simulink model "master_thesis_simulink"  (R2022a)
settings: Solver=VariableStepAuto  StartTime=0.0  StopTime=p_0p.time(end)  FixedStep=0.001  RelTol=1e-3
values from neighbouring files (symbols this model uses):
  markers_forearm = [0.00210510253906 -0.143263397217 -0.00798474121094]    [markers_forearm.mat]
  markers_shoulder = [0.010127746582 -0.151647644043 -0.0119686279297]    [markers_shoulder.mat]
undefined symbols (not defined in the file or in its folder): arm, DiscIntNeverNeededParam, Discrete, ekf, kf, LS, m, markers_hand, n, noise, q0, q0_LS, q0_model, sample_Time, selected, state_observer, Time, tSh_0_0Conf, X, Y, Z
libraries: sm_lib x2029, nesl_utility x1553, robotlib x75, ctrlSharedLib x8
(part 2 of 70)

== system master_thesis_simulink/System/Human arm ==
  note: B_shoulder
  note: SHOULDER
  note: ELBOW-FOREARM
  note: WRIST-HAND
  q ref : Inport
  Demux : Demux  Outputs=7
  Elbow_joint : Subsystem
      settings: PortSchema="{\"entries\":[{\"content\":{\"sides\":[{\"content\":{\"connectorIds\":[\"LConn1\",\"In1\"]},\"type\":\"ConnectorPlacement.EquallySpacedRectSide\",\"uuid\":\"7172d894-cd28-4181-98d4-69e790c9ffe7\"},{\"content\":{\"connectorIds\":[\"RConn1\"],\"side\":\"RIGHT\"},\"type\":\"ConnectorPlacement.EquallySpacedRectSide\",\"uuid\":\"72334abd-f6e9-45ab-9ec0-c8814621d72e\"},{\"content\":{\"connectorIds\":[],\"side\":\"TOP\"},\"type\":\"ConnectorPlacement.EquallySpacedRectSide\",\"uuid\":\"097d2b6b-6630-427f-97b0-bc88c7b983e5\"}]},\"type\":\"ConnectorPlacement.EquallySpacedConnector\",\"uuid\":\"52d59dae-be5f-4018-861b-6a79689710e1\"}],\"packageUris\":[\"http://schema.mathworks.com/mf0/Connector/R2020b\"],\"version\":\"1.0\"}"
  Markers : Subsystem  Commented=on
  Mechanism Configuration : sm_lib/Utilities/Mechanism Configuration  UniformGravity=Constant  GravityVector=[0 0 -9.80665]  GravityUnits=m/s^2  LinearizationDelta=0.001  JointModeTransitionNonlinearIterations=2
  Mux : Mux  Inputs=m
  Mux1 : Mux  Inputs=m
  Mux2 : Mux  Inputs=3
  Mux3 : Mux  Inputs=3
  RightForeArm : Subsystem
  RightHand : Subsystem
  RightShoulder : Subsystem
  RightShoulder_joint : Subsystem
      settings: PortSchema="{\"entries\":[{\"content\":{\"sides\":[{\"content\":{\"connectorIds\":[\"LConn1\",\"In1\"]},\"type\":\"ConnectorPlacement.EquallySpacedRectSide\",\"uuid\":\"7172d894-cd28-4181-98d4-69e790c9ffe7\"},{\"content\":{\"connectorIds\":[\"RConn1\"],\"side\":\"RIGHT\"},\"type\":\"ConnectorPlacement.EquallySpacedRectSide\",\"uuid\":\"72334abd-f6e9-45ab-9ec0-c8814621d72e\"},{\"content\":{\"connectorIds\":[],\"side\":\"TOP\"},\"type\":\"ConnectorPlacement.EquallySpacedRectSide\",\"uuid\":\"097d2b6b-6630-427f-97b0-bc88c7b983e5\"}]},\"type\":\"ConnectorPlacement.EquallySpacedConnector\",\"uuid\":\"52d59dae-be5f-4018-861b-6a79689710e1\"}],\"packageUris\":[\"http://schema.mathworks.com/mf0/Connector/R2020b\"],\"version\":\"1.0\"}"
  Solver Configuration1 : nesl_utility/Solver Configuration  PhysicalDomain=network_engine_domain  SubClassName=solver  LeftPortType=input  RightPortType=generic  Tones=[]  Harmonics=[]  SimulateNoise=off  Profile=off  UseLocalSampling=off  EnableSwitchedLinearOptims=on  FrequencyDomain=off  UseCCode=off  RelTol=0.001  AbsTol=0.001  MinStep=1e-09  ToWorkspace=off  RevertToSquareIcSolve=off  NumHomotopyIterations=100  PhasorMode=off  PhasorModeNumHarmonics=1  IndexReductionMethod=DerivativeReplacement  DoDC=off  ResidualTolerance=1e-09  UseLocalSolver=off  LocalSolverChoice=NE_BACKWARD_EULER_ADVANCER  LocalSolverSampleTime=0.001  DoFixedCost=off  MaxNonlinIter=3  MaxModeIter=2  ComputeImpulses=off  ImpulseIterations=2  LinearAlgebra=auto  LinearAlgebraNumThread=0  EquationFormulation=NE_TIME_EF  DelaysMemoryBudget=1024  AutomaticFiltering=on  FilteringTimeConstant=0.001  PartitionStorageMethod=AS_NEEDED  PartitionMemoryBudget=1024  PartitionMethod=ROBUST
      settings: SourceProductBaseCode=SS,PW,VE
  World Frame : sm_lib/Frames and Transforms/World Frame
  Wrist_joint : Subsystem
  p : Outport
  pdot : Outport  Port=2
  wires:
  Mux/1 -> p/1
  Mux1/1 -> pdot/1
  q ref/1 -> Demux/1
  Demux/7 -> Mux3/3
  Demux/1 -> Mux2/1
  Demux/2 -> Mux2/2
  Demux/3 -> Mux2/3
  Demux/6 -> Mux3/2
  Demux/5 -> Mux3/1
  Demux/4 -> [q_El]
  Mux2/1 -> [q_Sh]
  Mux3/1 -> [q_Wr]
  [q_Sh] -> RightShoulder_joint/1(q ref 1..3)
  [q_Wr] -> Wrist_joint/1(q ref 5..7)
  [q_El] -> Elbow_joint/1(q ref 4)
  [p_1] -> Mux/1
  [pdot_1] -> Mux1/1
  [p_2] -> Mux/2
  [pdot_2] -> Mux1/2
  [p_3] -> Mux/3
  [pdot_3] -> Mux1/3
  connections:
  RightShoulder/LConn1 -- RightShoulder_joint/RConn1
  RightHand/LConn1 -- Wrist_joint/RConn1
  Elbow_joint/LConn1 -- RightShoulder/RConn1
  RightForeArm/LConn2 -- RightHand/LConn2 -- RightShoulder/LConn2 -- World Frame/RConn1 -- RightShoulder_joint/LConn1 -- Mechanism Configuration/RConn1 -- Solver Configuration1/RConn1
  Elbow_joint/RConn1 -- RightForeArm/LConn1
  RightForeArm/RConn1 -- Wrist_joint/LConn1

== system master_thesis_simulink/System/LKF ==
  pdot_k : Inport
  p_k : Inport  Port=2
  Kalman Filter : MATLAB Function  TreatAsAtomicUnit=on
  Kalman Filter1 : ctrlSharedLib/Kalman Filter  Commented=on  TimeDomain=Discrete-Time  UseCurrentEstimator=on  ModelSource=Individual A, B, C, D matrices  ModelSourceVariable=ss(0.95,1,1,0,1)  A=kf.F  B=kf.G  C=kf.J  D=kf.I  NumberOfStates=1  NumberOfInputs=1  NumberOfOutputs=1  InitialEstimateSource=Dialog  X0=kf.Delta_q0  P0=kf.P0  UseK=off  UseGH=off  NumberOfProcessNoiseInputs=1  G=1  TimeInvariantG=on  H=0  TimeInvariantH=on  Q=noise.Q  TimeInvariantQ=on  R=noise.R  TimeInvariantR=on  N=0  TimeInvariantN=on  AddInputPort=on  AddEnablePort=off  OutputEstimatedY=off  OutputP=off  Ts=sample_Time
  Saturation : Saturate  UpperLimit=[pi/2; pi/10; 2/3*pi; pi/2; pi/4; pi/10; pi/4]  LowerLimit="[-pi/2; -pi/10; -pi/6; 0; -pi/2;  -pi/2; -pi/4]"
  Scope : Scope  NumInputPorts=2
  Sum2 : Sum  Inputs=++|
  Sum3 : Sum  Inputs=|+-
  Sum4 : Sum  Inputs=++|
  Sum6 : Sum  Inputs=|+-
  To Workspace1 : ToWorkspace  VariableName=q_KF  SaveFormat=Structure With Time  SampleTime=-1
  p_eq : Constant  Value=kf.p_eq  SampleTime=sample_Time
  pdot_eq : Constant  Value=kf.pdot_eq  SampleTime=sample_Time
  q_eq : Constant  Value=kf.q_eq  SampleTime=sample_Time
  q_eq1 : Constant  Value=kf.q_eq  SampleTime=sample_Time
  q_KF : Outport
  wires:
  pdot_k/1 -> Sum3/1
  pdot_eq/1 -> Sum3/2
  Sum3/1 -> Kalman Filter1/1, Kalman Filter/2(Delta_pdotk_1)
  Kalman Filter/1(Delta_qk) -> Sum2/2
  Kalman Filter1/1 -> Sum4/2
  q_eq1/1 -> Sum4/1
  Sum4/1 -> Scope/2  "kf simulink"
  p_k/1 -> Sum6/1
  p_eq/1 -> Sum6/2  "u_eqk"
  Sum6/1 -> Kalman Filter1/2, Kalman Filter/1(Delta_pk)  "Delta_uk"
  q_eq/1 -> Sum2/1
  Sum2/1 -> Saturation/1  "kf"
  Saturation/1 -> To Workspace1/1, q_KF/1, Scope/1

== system master_thesis_simulink/System/LS ==
  pdot : Inport
  Integrator : Integrator  InitialCondition=q0_LS  LimitOutput=on  UpperSaturationLimit=[pi/2; pi/10; 2/3*pi; pi/2; pi/4; pi/10; pi/4]  LowerSaturationLimit="[-pi/2; -pi/10; -pi/6; 0; -pi/2;  -pi/2; -pi/4]"
  LS : MATLAB Function  TreatAsAtomicUnit=on
  To Workspace1 : ToWorkspace  VariableName=q_LS_MinimumNorm  SaveFormat=Structure With Time  SampleTime=-1
  q_LS : Outport
  tag scope: q_LS_MinimumNorm=global
  wires:
  [markers_s] -> LS/3(shoulder_variables)
  [markers_h] -> LS/5(hand_variables)
  [markers_f] -> LS/4(forearm_variables)
  pdot/1 -> LS/2(pdot)
  [q_LS_MinimumNorm] -> LS/1(q_LS_MinimumNorm)
  Integrator/1 -> To Workspace1/1, q_LS/1, [q_LS_MinimumNorm]  "q_LS_MinimumNorm"
  LS/1(qdot_LS_MinimumNorm) -> Integrator/1

== system master_thesis_simulink/System/Noisy p ==
  p_true : Inport
  Sum1 : Sum  Inputs=++|
  v : RandomNumber  Variance=diag(noise.R)  Seed=2  SampleTime=sample_Time
  p : Outport
  wires:
  p_true/1 -> Sum1/2
  Sum1/1 -> p/1  "p"
  v/1 -> Sum1/1

== system master_thesis_simulink/System/Noisy pdot ==
  pdot_true : Inport
  Sum1 : Sum  Inputs=++|
  n_pdot : RandomNumber  Variance=diag(noise.N_pdot)  Seed=2  SampleTime=sample_Time
  pdot : Outport
  wires:
  pdot_true/1 -> Sum1/2
  Sum1/1 -> pdot/1  "pdot"
  n_pdot/1 -> Sum1/1

== system master_thesis_simulink/System/Show Results ==
  EKF : Subsystem
  From Workspace : FromWorkspace  VariableName=p_0p  SampleTime=-1
  From Workspace1 : FromWorkspace  VariableName=v_0p  SampleTime=-1
  KF : Subsystem
  LS : Subsystem
  Scope1 : Scope
  Scope3 : Scope
  Zero-Order Hold1 : ZeroOrderHold  SampleTime=sample_Time
  Zero-Order Hold4 : ZeroOrderHold  SampleTime=sample_Time
  tag scope: p_0p=global, v_0p=global
  wires:
  From Workspace1/1 -> Zero-Order Hold4/1
  From Workspace/1 -> Zero-Order Hold1/1
  Zero-Order Hold4/1 -> Scope3/1, [v_0p]  "p_noisyk"
  Zero-Order Hold1/1 -> Scope1/1, [p_0p]  "p_noisyk"

== system master_thesis_simulink/Experiments/S0_F1_H2/Experiments ==
  p_0' : Inport
  v_0' : Inport  Port=2
  Selector : Inport  Port=3
  Action Port : ActionPort  ActionPortLabel=if(u1 > 0)
  Constant : Constant  Value=markers_shoulder
  Constant1 : Constant  Value=markers_forearm
  Constant2 : Constant  Value=markers_hand
  EKF : Subsystem
  Human arm : Subsystem  Commented=on
  Human arm_exp : Subsystem  Commented=on
  KF : Subsystem  Commented=on
  LS : Subsystem  Commented=on
  Switch Case : SwitchCase  CaseConditions={0, 1, 2, -1}  ShowDefaultCase=off
  Terminator : Terminator
  tag scope: markers_fo=global, markers_ha=global, markers_sh=global
  wires:
  p_0'/1 -> LS/1(p_0'), EKF/1(p_0'), KF/1(p_0')
  v_0'/1 -> KF/2(v_0'), EKF/2(v_0'), LS/2(v_0')
  Switch Case/1 -> LS/Action
  Switch Case/2 -> KF/Action
  Selector/1 -> Switch Case/1
  [markers_fo] -> LS/4(markers forearm)
  [markers_ha] -> LS/5(markers hand)
  [markers_sh] -> LS/3(markers shoulder)
  [markers_fo] -> EKF/4(markers forearm)
  [markers_ha] -> EKF/5(markers hand)
  [markers_sh] -> EKF/3(markers shoulder)
  Switch Case/4 -> Terminator/1
  Switch Case/3 -> EKF/Action
  Constant1/1 -> [markers_fo]
  Constant/1 -> [markers_sh]
  Constant2/1 -> [markers_ha]

== system master_thesis_simulink/Experiments/S0_F1_H2/Model validation ==
  p_0' : Inport
  Action Port : ActionPort  ActionPortLabel=if(u1 > 0)
  Average : MATLAB Function  TreatAsAtomicUnit=on
  Constant : Constant  Value=zeros(7, 1)
  Display : Subsystem
  Human arm : Subsystem  Commented=on
  Markers_Bases : MATLAB Function  TreatAsAtomicUnit=on
  Mux : Mux  Inputs=3
  Reshape : Reshape  OutputDimensionality=Column vector (2-D)
  Scope : Scope
  To Workspace : ToWorkspace  VariableName=markers_Bases  SaveFormat=Structure With Time  SampleTime=-1
  p_0'1 : InportShadow
  p_v__vs_FK_J : MATLAB Function  TreatAsAtomicUnit=on
  wires:
  Markers_Bases/1(markers_shoulder) -> Mux/1, p_v__vs_FK_J/2(shoulder_variables)
  Markers_Bases/2(markers_forearm) -> p_v__vs_FK_J/3(forearm_variables), Mux/2
  Markers_Bases/3(markers_hand) -> Reshape/1, p_v__vs_FK_J/4(hand_variables)
  Constant/1 -> p_v__vs_FK_J/1(q)
  p_0'/1 -> Display/1(p_0')
  Mux/1 -> Scope/1, To Workspace/1
  p_v__vs_FK_J/1(p_Model) -> Display/2(p_FK)
  Reshape/1 -> Mux/3
  Average/1(pk_hat) -> Markers_Bases/1(p_0p_mean)
  p_0'1/1 -> Average/1(pk)

== system master_thesis_simulink/Experiments/S0_F1_H2/Noise estimation ==
  Rp0_W : Inport
  Rpi_W : Inport  Port=2
  Rv0_W : Inport  Port=3
  Rvi_W : Inport  Port=4
  Action Port : ActionPort  ActionPortLabel=if(u1 > 0)
  Average : MATLAB Function  TreatAsAtomicUnit=on
  Noise Covariance of pi_0 Average : MATLAB Function  TreatAsAtomicUnit=on
  Noise Covariance of vi_0 Average : MATLAB Function  TreatAsAtomicUnit=on
  Selector1 : Selector  NumberOfDimensions=2  InputPortWidth=3  IndexOptions=Index vector (dialog),Index vector (dialog)  Indices=1:3,1:3  OutputSizes=1,1
  Selector2 : Selector  NumberOfDimensions=2  InputPortWidth=3  IndexOptions=Index vector (dialog),Index vector (dialog)  Indices=4:6,1:3  OutputSizes=1,1
  Selector3 : Selector  NumberOfDimensions=2  InputPortWidth=3  IndexOptions=Index vector (dialog),Index vector (dialog)  Indices=7:9,1:3  OutputSizes=1,1
  Selector4 : Selector  NumberOfDimensions=2  InputPortWidth=3  IndexOptions=Index vector (dialog),Index vector (dialog)  Indices=1:3,1:3  OutputSizes=1,1
  Selector5 : Selector  NumberOfDimensions=2  InputPortWidth=3  IndexOptions=Index vector (dialog),Index vector (dialog)  Indices=4:6,1:3  OutputSizes=1,1
  Selector6 : Selector  NumberOfDimensions=2  InputPortWidth=3  IndexOptions=Index vector (dialog),Index vector (dialog)  Indices=7:9,1:3  OutputSizes=1,1
  To Workspace : ToWorkspace  VariableName=Rp1_0p  SaveFormat=Structure With Time  SampleTime=-1
  To Workspace1 : ToWorkspace  VariableName=Rp2_0p  SaveFormat=Structure With Time  SampleTime=-1
  To Workspace2 : ToWorkspace  VariableName=Rp3_0p  SaveFormat=Structure With Time  SampleTime=-1
  To Workspace4 : ToWorkspace  VariableName=Rv1_0p  SaveFormat=Structure With Time  SampleTime=-1
  To Workspace5 : ToWorkspace  VariableName=Rv2_0p  SaveFormat=Structure With Time  SampleTime=-1
  To Workspace6 : ToWorkspace  VariableName=Rv3_0p  SaveFormat=Structure With Time  SampleTime=-1
  wires:
  Rp0_W/1 -> Average/1(Rp0_W)
  Rpi_W/1 -> Average/2(Rpi_W)
  Noise Covariance of pi_0 Average/1(Rk_hat) -> Selector4/1, Selector5/1, Selector6/1
  Average/1(Rpi_0p) -> Noise Covariance of pi_0 Average/1(Rk)
  Selector4/1 -> To Workspace/1
  Selector5/1 -> To Workspace1/1
  Selector6/1 -> To Workspace2/1
  Rvi_W/1 -> Average/4(Rvi_W)
  Rv0_W/1 -> Average/3(Rv0_W)
  Average/2(Rvi_0p) -> Noise Covariance of vi_0 Average/1(Rk)
  Selector3/1 -> To Workspace6/1
  Selector2/1 -> To Workspace5/1
  Selector1/1 -> To Workspace4/1
  Noise Covariance of vi_0 Average/1(Rk_hat) -> Selector1/1, Selector2/1, Selector3/1

== system master_thesis_simulink/Experiments/S0_F2_H2/Experiments ==
  p_0' : Inport
  v_0' : Inport  Port=2
  Selector : Inport  Port=3
  Action Port : ActionPort  ActionPortLabel=if(u1 > 0)
  Constant : Constant  Value=markers_shoulder
  Constant1 : Constant  Value=markers_forearm
  Constant2 : Constant  Value=markers_hand
  EKF : Subsystem
  Human arm : Subsystem  Commented=on
  Human arm_exp : Subsystem  Commented=on
  KF : Subsystem  Commented=on
  LS : Subsystem  Commented=on
  Switch Case : SwitchCase  CaseConditions={0, 1, 2, -1}  ShowDefaultCase=off
  Terminator : Terminator
  tag scope: markers_fo=global, markers_ha=global, markers_sh=global
  wires:
  Constant2/1 -> [markers_ha]
  Constant/1 -> [markers_sh]
  Constant1/1 -> [markers_fo]
  Switch Case/3 -> EKF/Action
  Switch Case/4 -> Terminator/1
  [markers_sh] -> EKF/3(markers shoulder)
  [markers_ha] -> EKF/5(markers hand)
  [markers_fo] -> EKF/4(markers forearm)
  [markers_sh] -> LS/3(markers shoulder)
  [markers_ha] -> LS/5(markers hand)
  [markers_fo] -> LS/4(markers forearm)
  Selector/1 -> Switch Case/1
  Switch Case/2 -> KF/Action
  Switch Case/1 -> LS/Action
  v_0'/1 -> LS/2(v_0'), EKF/2(v_0'), KF/2(v_0')
  p_0'/1 -> KF/1(p_0'), EKF/1(p_0'), LS/1(p_0')

== system master_thesis_simulink/Experiments/S0_F2_H2/Model validation ==
  p_0' : Inport
  Action Port : ActionPort  ActionPortLabel=if(u1 > 0)
  Average : MATLAB Function  TreatAsAtomicUnit=on
  Constant : Constant  Value=zeros(7, 1)
  Display : Subsystem
  Human arm : Subsystem  Commented=on
  Markers_Bases : MATLAB Function  TreatAsAtomicUnit=on
  Mux : Mux  Inputs=3
  Reshape : Reshape  OutputDimensionality=Column vector (2-D)
  Reshape1 : Reshape  OutputDimensionality=Column vector (2-D)
  Scope : Scope
  To Workspace : ToWorkspace  VariableName=markers_Bases  SaveFormat=Structure With Time  SampleTime=-1
  p_0'1 : InportShadow
  p_v__vs_FK_J : MATLAB Function  TreatAsAtomicUnit=on
  wires:
  p_0'1/1 -> Average/1(pk)
  Average/1(pk_hat) -> Markers_Bases/1(p_0p_mean)
  Reshape/1 -> Mux/3
  p_v__vs_FK_J/1(p_Model) -> Display/2(p_FK)
  Mux/1 -> To Workspace/1, Scope/1
  p_0'/1 -> Display/1(p_0')
  Constant/1 -> p_v__vs_FK_J/1(q)
  Markers_Bases/3(markers_hand) -> p_v__vs_FK_J/4(hand_variables), Reshape/1
  Markers_Bases/2(markers_forearm) -> p_v__vs_FK_J/3(forearm_variables), Reshape1/1
  Markers_Bases/1(markers_shoulder) -> p_v__vs_FK_J/2(shoulder_variables), Mux/1
  Reshape1/1 -> Mux/2

== system master_thesis_simulink/Experiments/S0_F2_H2/Noise estimation ==
  Rp0_W : Inport
  Rpi_W : Inport  Port=2
  Rv0_W : Inport  Port=3
  Rvi_W : Inport  Port=4
  Action Port : ActionPort  ActionPortLabel=if(u1 > 0)
  Average : MATLAB Function  TreatAsAtomicUnit=on
  Noise Covariance of pi_0 Average : MATLAB Function  TreatAsAtomicUnit=on
  Noise Covariance of vi_0 Average : MATLAB Function  TreatAsAtomicUnit=on
  Selector1 : Selector  NumberOfDimensions=2  InputPortWidth=3  IndexOptions=Index vector (dialog),Index vector (dialog)  Indices=1:3,1:3  OutputSizes=1,1
  Selector2 : Selector  NumberOfDimensions=2  InputPortWidth=3  IndexOptions=Index vector (dialog),Index vector (dialog)  Indices=4:6,1:3  OutputSizes=1,1
  Selector3 : Selector  NumberOfDimensions=2  InputPortWidth=3  IndexOptions=Index vector (dialog),Index vector (dialog)  Indices=7:9,1:3  OutputSizes=1,1
  Selector4 : Selector  NumberOfDimensions=2  InputPortWidth=3  IndexOptions=Index vector (dialog),Index vector (dialog)  Indices=1:3,1:3  OutputSizes=1,1
  Selector5 : Selector  NumberOfDimensions=2  InputPortWidth=3  IndexOptions=Index vector (dialog),Index vector (dialog)  Indices=4:6,1:3  OutputSizes=1,1
  Selector6 : Selector  NumberOfDimensions=2  InputPortWidth=3  IndexOptions=Index vector (dialog),Index vector (dialog)  Indices=7:9,1:3  OutputSizes=1,1
  Selector7 : Selector  NumberOfDimensions=2  InputPortWidth=3  IndexOptions=Index vector (dialog),Index vector (dialog)  Indices=10:12,1:3  OutputSizes=1,1
  Selector8 : Selector  NumberOfDimensions=2  InputPortWidth=3  IndexOptions=Index vector (dialog),Index vector (dialog)  Indices=10:12,1:3  OutputSizes=1,1
  To Workspace : ToWorkspace  VariableName=Rp1_0p  SaveFormat=Structure With Time  SampleTime=-1
  To Workspace1 : ToWorkspace  VariableName=Rp2_0p  SaveFormat=Structure With Time  SampleTime=-1
  To Workspace2 : ToWorkspace  VariableName=Rp3_0p  SaveFormat=Structure With Time  SampleTime=-1
  To Workspace3 : ToWorkspace  VariableName=Rp4_0p  SaveFormat=Structure With Time  SampleTime=-1
  To Workspace4 : ToWorkspace  VariableName=Rv1_0p  SaveFormat=Structure With Time  SampleTime=-1
  To Workspace5 : ToWorkspace  VariableName=Rv2_0p  SaveFormat=Structure With Time  SampleTime=-1
  To Workspace6 : ToWorkspace  VariableName=Rv3_0p  SaveFormat=Structure With Time  SampleTime=-1
  To Workspace7 : ToWorkspace  VariableName=Rv4_0p  SaveFormat=Structure With Time  SampleTime=-1
  wires:
  Noise Covariance of vi_0 Average/1(Rk_hat) -> Selector8/1, Selector3/1, Selector2/1, Selector1/1
  Selector1/1 -> To Workspace4/1
  Selector2/1 -> To Workspace5/1
  Selector3/1 -> To Workspace6/1
  Selector8/1 -> To Workspace7/1
  Average/2(Rvi_0p) -> Noise Covariance of vi_0 Average/1(Rk)
  Rv0_W/1 -> Average/3(Rv0_W)
  Rvi_W/1 -> Average/4(Rvi_W)
  Selector7/1 -> To Workspace3/1
  Selector6/1 -> To Workspace2/1
  Selector5/1 -> To Workspace1/1
  Selector4/1 -> To Workspace/1
  Average/1(Rpi_0p) -> Noise Covariance of pi_0 Average/1(Rk)
  Noise Covariance of pi_0 Average/1(Rk_hat) -> Selector7/1, Selector6/1, Selector5/1, Selector4/1
  Rpi_W/1 -> Average/2(Rpi_W)
  Rp0_W/1 -> Average/1(Rp0_W)

== system master_thesis_simulink/Experiments/S1_F0_H2/Experiments ==
  p_0' : Inport
  v_0' : Inport  Port=2
  Selector : Inport  Port=3
  Action Port : ActionPort  ActionPortLabel=if(u1 > 0)
  Constant : Constant  Value=markers_shoulder
  Constant1 : Constant  Value=markers_forearm
  Constant2 : Constant  Value=markers_hand
  EKF : Subsystem
  Human arm : Subsystem  Commented=on
  Human arm_exp : Subsystem  Commented=on
  KF : Subsystem  Commented=on
  LS : Subsystem  Commented=on
  Switch Case : SwitchCase  CaseConditions={0, 1, 2, -1}  ShowDefaultCase=off
  Terminator : Terminator
  tag scope: markers_fo=global, markers_ha=global, markers_sh=global
  wires:
  p_0'/1 -> LS/1(p_0'), EKF/1(p_0'), KF/1(p_0')
  v_0'/1 -> KF/2(v_0'), EKF/2(v_0'), LS/2(v_0')
  Switch Case/1 -> LS/Action
  Switch Case/2 -> KF/Action
  Selector/1 -> Switch Case/1
  [markers_fo] -> LS/4(markers forearm)
  [markers_ha] -> LS/5(markers hand)
  [markers_sh] -> LS/3(markers shoulder)
  [markers_fo] -> EKF/4(markers forearm)
  [markers_ha] -> EKF/5(markers hand)
  [markers_sh] -> EKF/3(markers shoulder)
  Switch Case/4 -> Terminator/1
  Switch Case/3 -> EKF/Action
  Constant1/1 -> [markers_fo]
  Constant/1 -> [markers_sh]
  Constant2/1 -> [markers_ha]

== system master_thesis_simulink/Experiments/S1_F0_H2/Model validation ==
  p_0' : Inport
  Action Port : ActionPort  ActionPortLabel=if(u1 > 0)
  Average : MATLAB Function  TreatAsAtomicUnit=on
  Constant : Constant  Value=zeros(7, 1)
  Display : Subsystem
  Human arm : Subsystem  Commented=on
  Markers_Bases : MATLAB Function  TreatAsAtomicUnit=on
  Mux : Mux  Inputs=3
  Reshape : Reshape  OutputDimensionality=Column vector (2-D)
  Scope : Scope
  To Workspace : ToWorkspace  VariableName=markers_Bases  SaveFormat=Structure With Time  SampleTime=-1
  p_0'1 : InportShadow
  p_v__vs_FK_J : MATLAB Function  TreatAsAtomicUnit=on
  wires:
  Markers_Bases/1(markers_shoulder) -> Mux/1, p_v__vs_FK_J/2(shoulder_variables)
  Markers_Bases/2(markers_forearm) -> p_v__vs_FK_J/3(forearm_variables), Mux/2
  Markers_Bases/3(markers_hand) -> Reshape/1, p_v__vs_FK_J/4(hand_variables)
  Constant/1 -> p_v__vs_FK_J/1(q)
  p_0'/1 -> Display/1(p_0')
  Mux/1 -> Scope/1, To Workspace/1
  p_v__vs_FK_J/1(p_Model) -> Display/2(p_FK)
  Reshape/1 -> Mux/3
  Average/1(pk_hat) -> Markers_Bases/1(p_0p_mean)
  p_0'1/1 -> Average/1(pk)

== system master_thesis_simulink/Experiments/S1_F0_H2/Noise estimation ==
  Rp0_W : Inport
  Rpi_W : Inport  Port=2
  Rv0_W : Inport  Port=3
  Rvi_W : Inport  Port=4
  Action Port : ActionPort  ActionPortLabel=if(u1 > 0)
  Average : MATLAB Function  TreatAsAtomicUnit=on
  Noise Covariance of pi_0 Average : MATLAB Function  TreatAsAtomicUnit=on
  Noise Covariance of vi_0 Average : MATLAB Function  TreatAsAtomicUnit=on
  Selector1 : Selector  NumberOfDimensions=2  InputPortWidth=3  IndexOptions=Index vector (dialog),Index vector (dialog)  Indices=1:3,1:3  OutputSizes=1,1
  Selector2 : Selector  NumberOfDimensions=2  InputPortWidth=3  IndexOptions=Index vector (dialog),Index vector (dialog)  Indices=4:6,1:3  OutputSizes=1,1
  Selector3 : Selector  NumberOfDimensions=2  InputPortWidth=3  IndexOptions=Index vector (dialog),Index vector (dialog)  Indices=7:9,1:3  OutputSizes=1,1
  Selector4 : Selector  NumberOfDimensions=2  InputPortWidth=3  IndexOptions=Index vector (dialog),Index vector (dialog)  Indices=1:3,1:3  OutputSizes=1,1
  Selector5 : Selector  NumberOfDimensions=2  InputPortWidth=3  IndexOptions=Index vector (dialog),Index vector (dialog)  Indices=4:6,1:3  OutputSizes=1,1
  Selector6 : Selector  NumberOfDimensions=2  InputPortWidth=3  IndexOptions=Index vector (dialog),Index vector (dialog)  Indices=7:9,1:3  OutputSizes=1,1
  To Workspace : ToWorkspace  VariableName=Rp1_0p  SaveFormat=Structure With Time  SampleTime=-1
  To Workspace1 : ToWorkspace  VariableName=Rp2_0p  SaveFormat=Structure With Time  SampleTime=-1
  To Workspace2 : ToWorkspace  VariableName=Rp3_0p  SaveFormat=Structure With Time  SampleTime=-1
  To Workspace4 : ToWorkspace  VariableName=Rv1_0p  SaveFormat=Structure With Time  SampleTime=-1
  To Workspace5 : ToWorkspace  VariableName=Rv2_0p  SaveFormat=Structure With Time  SampleTime=-1
  To Workspace6 : ToWorkspace  VariableName=Rv3_0p  SaveFormat=Structure With Time  SampleTime=-1
  wires:
  Rp0_W/1 -> Average/1(Rp0_W)
  Rpi_W/1 -> Average/2(Rpi_W)
  Noise Covariance of pi_0 Average/1(Rk_hat) -> Selector4/1, Selector5/1, Selector6/1
  Average/1(Rpi_0p) -> Noise Covariance of pi_0 Average/1(Rk)
  Selector4/1 -> To Workspace/1
  Selector5/1 -> To Workspace1/1
  Selector6/1 -> To Workspace2/1
  Rvi_W/1 -> Average/4(Rvi_W)
  Rv0_W/1 -> Average/3(Rv0_W)
  Average/2(Rvi_0p) -> Noise Covariance of vi_0 Average/1(Rk)
  Selector3/1 -> To Workspace6/1
  Selector2/1 -> To Workspace5/1
  Selector1/1 -> To Workspace4/1
  Noise Covariance of vi_0 Average/1(Rk_hat) -> Selector1/1, Selector2/1, Selector3/1

== system master_thesis_simulink/Experiments/S1_F0_H3/Experiments ==
  p_0' : Inport
  v_0' : Inport  Port=2
  Selector : Inport  Port=3
  Action Port : ActionPort
  Constant : Constant  Value=markers_shoulder
  Constant1 : Constant  Value=markers_forearm
  Constant2 : Constant  Value=markers_hand
  EKF : Subsystem
  Human arm : Subsystem  Commented=on
  Human arm_exp : Subsystem  Commented=on
  KF : Subsystem  Commented=on
  LS : Subsystem  Commented=on
  Switch Case : SwitchCase  CaseConditions={0, 1, 2, -1}  ShowDefaultCase=off
  Terminator : Terminator
  tag scope: markers_fo=global, markers_ha=global, markers_sh=global
  wires:
  p_0'/1 -> LS/1(p_0'), EKF/1(p_0'), KF/1(p_0')
  v_0'/1 -> KF/2(v_0'), EKF/2(v_0'), LS/2(v_0')
  Switch Case/1 -> LS/Action
  Switch Case/2 -> KF/Action
  Selector/1 -> Switch Case/1
  [markers_fo] -> LS/4(markers forearm)
  [markers_ha] -> LS/5(markers hand)
  [markers_sh] -> LS/3(markers shoulder)
  [markers_fo] -> EKF/4(markers forearm)
  [markers_ha] -> EKF/5(markers hand)
  [markers_sh] -> EKF/3(markers shoulder)
  Switch Case/4 -> Terminator/1
  Switch Case/3 -> EKF/Action
  Constant1/1 -> [markers_fo]
  Constant/1 -> [markers_sh]
  Constant2/1 -> [markers_ha]

== system master_thesis_simulink/Experiments/S1_F0_H3/Model validation ==
  p_0' : Inport
  Action Port : ActionPort  ActionPortLabel=if(u1 > 0)
  Average : MATLAB Function  TreatAsAtomicUnit=on
  Constant : Constant  Value=zeros(7, 1)
  Display : Subsystem
  Human arm : Subsystem  Commented=on
  Markers_Bases : MATLAB Function  TreatAsAtomicUnit=on
  Mux : Mux  Inputs=3
  Reshape : Reshape  OutputDimensionality=Column vector (2-D)
  Scope : Scope
  To Workspace : ToWorkspace  VariableName=markers_Bases  SaveFormat=Structure With Time  SampleTime=-1
  p_0'1 : InportShadow
  p_v__vs_FK_J : MATLAB Function  TreatAsAtomicUnit=on
  wires:
  Markers_Bases/1(markers_shoulder) -> Mux/1, p_v__vs_FK_J/2(shoulder_variables)
  Markers_Bases/2(markers_forearm) -> p_v__vs_FK_J/3(forearm_variables), Mux/2
  Markers_Bases/3(markers_hand) -> Reshape/1, p_v__vs_FK_J/4(hand_variables)
  Constant/1 -> p_v__vs_FK_J/1(q)
  p_0'/1 -> Display/1(p_0')
  Mux/1 -> Scope/1, To Workspace/1
  p_v__vs_FK_J/1(p_Model) -> Display/2(p_FK)
  Reshape/1 -> Mux/3
  Average/1(pk_hat) -> Markers_Bases/1(p_0p_mean)
  p_0'1/1 -> Average/1(pk)

== system master_thesis_simulink/Experiments/S1_F0_H3/Noise estimation ==
  Rp0_W : Inport
  Rpi_W : Inport  Port=2
  Rv0_W : Inport  Port=3
  Rvi_W : Inport  Port=4
  Action Port : ActionPort  ActionPortLabel=if(u1 > 0)
  Average : MATLAB Function  TreatAsAtomicUnit=on
  Noise Covariance of pi_0 Average : MATLAB Function  TreatAsAtomicUnit=on
  Noise Covariance of vi_0 Average : MATLAB Function  TreatAsAtomicUnit=on
  Selector1 : Selector  NumberOfDimensions=2  InputPortWidth=3  IndexOptions=Index vector (dialog),Index vector (dialog)  Indices=1:3,1:3  OutputSizes=1,1
  Selector2 : Selector  NumberOfDimensions=2  InputPortWidth=3  IndexOptions=Index vector (dialog),Index vector (dialog)  Indices=4:6,1:3  OutputSizes=1,1
  Selector3 : Selector  NumberOfDimensions=2  InputPortWidth=3  IndexOptions=Index vector (dialog),Index vector (dialog)  Indices=7:9,1:3  OutputSizes=1,1
  Selector4 : Selector  NumberOfDimensions=2  InputPortWidth=3  IndexOptions=Index vector (dialog),Index vector (dialog)  Indices=1:3,1:3  OutputSizes=1,1
  Selector5 : Selector  NumberOfDimensions=2  InputPortWidth=3  IndexOptions=Index vector (dialog),Index vector (dialog)  Indices=4:6,1:3  OutputSizes=1,1
  Selector6 : Selector  NumberOfDimensions=2  InputPortWidth=3  IndexOptions=Index vector (dialog),Index vector (dialog)  Indices=7:9,1:3  OutputSizes=1,1
  Selector7 : Selector  NumberOfDimensions=2  InputPortWidth=3  IndexOptions=Index vector (dialog),Index vector (dialog)  Indices=10:12,1:3  OutputSizes=1,1
  Selector8 : Selector  NumberOfDimensions=2  InputPortWidth=3  IndexOptions=Index vector (dialog),Index vector (dialog)  Indices=10:12,1:3  OutputSizes=1,1
  To Workspace : ToWorkspace  VariableName=Rp1_0p  SaveFormat=Structure With Time  SampleTime=-1
  To Workspace1 : ToWorkspace  VariableName=Rp2_0p  SaveFormat=Structure With Time  SampleTime=-1
  To Workspace2 : ToWorkspace  VariableName=Rp3_0p  SaveFormat=Structure With Time  SampleTime=-1
  To Workspace3 : ToWorkspace  VariableName=Rp4_0p  SaveFormat=Structure With Time  SampleTime=-1
  To Workspace4 : ToWorkspace  VariableName=Rv1_0p  SaveFormat=Structure With Time  SampleTime=-1
  To Workspace5 : ToWorkspace  VariableName=Rv2_0p  SaveFormat=Structure With Time  SampleTime=-1
  To Workspace6 : ToWorkspace  VariableName=Rv3_0p  SaveFormat=Structure With Time  SampleTime=-1
  To Workspace7 : ToWorkspace  VariableName=Rv4_0p  SaveFormat=Structure With Time  SampleTime=-1
  wires:
  Rp0_W/1 -> Average/1(Rp0_W)
  Rpi_W/1 -> Average/2(Rpi_W)
  Noise Covariance of pi_0 Average/1(Rk_hat) -> Selector4/1, Selector5/1, Selector6/1, Selector7/1
  Average/1(Rpi_0p) -> Noise Covariance of pi_0 Average/1(Rk)
  Selector4/1 -> To Workspace/1
  Selector5/1 -> To Workspace1/1
  Selector6/1 -> To Workspace2/1
  Selector7/1 -> To Workspace3/1
  Rvi_W/1 -> Average/4(Rvi_W)
  Rv0_W/1 -> Average/3(Rv0_W)
  Average/2(Rvi_0p) -> Noise Covariance of vi_0 Average/1(Rk)
  Selector8/1 -> To Workspace7/1
  Selector3/1 -> To Workspace6/1
  Selector2/1 -> To Workspace5/1
  Selector1/1 -> To Workspace4/1
  Noise Covariance of vi_0 Average/1(Rk_hat) -> Selector1/1, Selector2/1, Selector3/1, Selector8/1

== system master_thesis_simulink/Experiments/S1_F1_H2/Experiments ==
  p_0' : Inport
  v_0' : Inport  Port=2
  Selector : Inport  Port=3
  Action Port : ActionPort  ActionPortLabel=if(u1 > 0)
  Constant : Constant  Value=markers_shoulder
  Constant1 : Constant  Value=markers_forearm
  Constant2 : Constant  Value=markers_hand
  EKF : Subsystem
  Human arm : Subsystem  Commented=on
  Human arm_exp : Subsystem  Commented=on
  KF : Subsystem  Commented=on
  LS : Subsystem  Commented=on
  Switch Case : SwitchCase  CaseConditions={0, 1, 2, -1}  ShowDefaultCase=off
  Terminator : Terminator
  Output : Outport
  tag scope: markers_fo=global, markers_ha=global, markers_sh=global
  wires:
  p_0'/1 -> LS/1(p_0'), EKF/1(p_0'), KF/1(p_0')
  v_0'/1 -> KF/2(v_0'), EKF/2(v_0'), LS/2(v_0')
  Switch Case/1 -> LS/Action
  Switch Case/2 -> KF/Action
  Selector/1 -> Switch Case/1
  [markers_fo] -> LS/4(markers forearm)
  [markers_ha] -> LS/5(markers hand)
  [markers_sh] -> LS/3(markers shoulder)
  [markers_fo] -> EKF/4(markers forearm)
  [markers_ha] -> EKF/5(markers hand)
  [markers_sh] -> EKF/3(markers shoulder)
  Switch Case/4 -> Terminator/1
  Switch Case/3 -> EKF/Action
  Constant1/1 -> [markers_fo]
  Constant/1 -> [markers_sh]
  Constant2/1 -> [markers_ha]
  EKF/1(Output) -> Output/1  "p_0'"

== system master_thesis_simulink/Experiments/S1_F1_H2/Human arm1 ==
  note: B_shoulder
  note: SHOULDER
  note: ELBOW-FOREARM
  note: WRIST-HAND
  q_EKF : Inport
  Demux : Demux  Outputs=7
  Elbow_joint : Subsystem
  Markers : Subsystem  Commented=on
  Mechanism Configuration : sm_lib/Utilities/Mechanism Configuration  UniformGravity=Constant  GravityVector=[0 0 -9.80665]  GravityUnits=m/s^2  LinearizationDelta=0.001  JointModeTransitionNonlinearIterations=2
  Mux2 : Mux  Inputs=3
  Mux3 : Mux  Inputs=3
  RightForeArm : Subsystem
  RightHand : Subsystem
  RightShoulder : Subsystem
  RightShoulder_joint : Subsystem
  Solver Configuration1 : nesl_utility/Solver Configuration  PhysicalDomain=network_engine_domain  SubClassName=solver  LeftPortType=input  RightPortType=generic  Tones=[]  Harmonics=[]  SimulateNoise=off  Profile=off  UseLocalSampling=off  EnableSwitchedLinearOptims=on  FrequencyDomain=off  UseCCode=off  RelTol=0.001  AbsTol=0.001  MinStep=1e-09  ToWorkspace=off  RevertToSquareIcSolve=off  NumHomotopyIterations=100  PhasorMode=off  PhasorModeNumHarmonics=1  IndexReductionMethod=DerivativeReplacement  DoDC=off  ResidualTolerance=1e-09  UseLocalSolver=off  LocalSolverChoice=NE_TRAPEZOIDAL_ADVANCER  LocalSolverSampleTime=0.01  DoFixedCost=off  MaxNonlinIter=3  MaxModeIter=2  ComputeImpulses=off  ImpulseIterations=2  LinearAlgebra=auto  LinearAlgebraNumThread=0  EquationFormulation=NE_TIME_EF  DelaysMemoryBudget=1024  AutomaticFiltering=on  FilteringTimeConstant=0.001  PartitionStorageMethod=AS_NEEDED  PartitionMemoryBudget=1024  PartitionMethod=ROBUST
      settings: SourceProductBaseCode=SS,PW,VE
  World Frame : sm_lib/Frames and Transforms/World Frame
  Wrist_joint : Subsystem
  wires:
  q_EKF/1 -> Demux/1
  Demux/1 -> Mux2/1
  Demux/2 -> Mux2/2
  Demux/3 -> Mux2/3
  Mux2/1 -> [q_sh]
  Demux/4 -> [q_fo]
  Mux3/1 -> [q_ha]
  Demux/7 -> Mux3/3
  Demux/6 -> Mux3/2
  Demux/5 -> Mux3/1
  [q_sh] -> RightShoulder_joint/1(Input)
  [q_fo] -> Elbow_joint/1(Input)
  [q_ha] -> Wrist_joint/1(Input)
  connections:
  RightShoulder/LConn1 -- RightShoulder_joint/RConn1
  RightHand/LConn1 -- Wrist_joint/RConn1
  Elbow_joint/LConn1 -- RightShoulder/RConn1
  Wrist_joint/LConn1 -- RightForeArm/RConn1
  RightForeArm/LConn2 -- RightHand/LConn2 -- RightShoulder/LConn2 -- World Frame/RConn1 -- Mechanism Configuration/RConn1 -- RightShoulder_joint/LConn1 -- Solver Configuration1/RConn1
  Elbow_joint/RConn1 -- RightForeArm/LConn1

== system master_thesis_simulink/Experiments/S1_F1_H2/Model validation ==
  p_0' : Inport
  Action Port : ActionPort  ActionPortLabel=if(u1 > 0)
  Average : MATLAB Function  TreatAsAtomicUnit=on
  Constant : Constant  Value=zeros(7, 1)
  Display : Subsystem
  Human arm : Subsystem  Commented=on
  Markers_Bases : MATLAB Function  TreatAsAtomicUnit=on
  Mux : Mux  Inputs=3
  Reshape : Reshape  OutputDimensionality=Column vector (2-D)
  Scope : Scope
  To Workspace : ToWorkspace  VariableName=markers_Bases  SaveFormat=Structure With Time  SampleTime=-1
  p_0'1 : InportShadow
  p_v__vs_FK_J : MATLAB Function  TreatAsAtomicUnit=on
  wires:
  Markers_Bases/1(markers_shoulder) -> Mux/1, p_v__vs_FK_J/2(shoulder_variables)
  Markers_Bases/2(markers_forearm) -> p_v__vs_FK_J/3(forearm_variables), Mux/2
  Markers_Bases/3(markers_hand) -> Reshape/1, p_v__vs_FK_J/4(hand_variables)
  Constant/1 -> p_v__vs_FK_J/1(q)
  p_0'/1 -> Display/1(p_0')
  Mux/1 -> Scope/1, To Workspace/1
  p_v__vs_FK_J/1(p_Model) -> Display/2(p_FK)
  Reshape/1 -> Mux/3
  Average/1(pk_hat) -> Markers_Bases/1(p_0p_mean)
  p_0'1/1 -> Average/1(pk)

== system master_thesis_simulink/Experiments/S1_F1_H2/Noise estimation ==
  Rp0_W : Inport
  Rpi_W : Inport  Port=2
  Rv0_W : Inport  Port=3
  Rvi_W : Inport  Port=4
  Action Port : ActionPort  ActionPortLabel=if(u1 > 0)
  Average : MATLAB Function  TreatAsAtomicUnit=on
  Noise Covariance of pi_0 Average : MATLAB Function  TreatAsAtomicUnit=on
  Noise Covariance of vi_0 Average : MATLAB Function  TreatAsAtomicUnit=on
  Selector1 : Selector  NumberOfDimensions=2  InputPortWidth=3  IndexOptions=Index vector (dialog),Index vector (dialog)  Indices=1:3,1:3  OutputSizes=1,1
  Selector2 : Selector  NumberOfDimensions=2  InputPortWidth=3  IndexOptions=Index vector (dialog),Index vector (dialog)  Indices=4:6,1:3  OutputSizes=1,1
  Selector3 : Selector  NumberOfDimensions=2  InputPortWidth=3  IndexOptions=Index vector (dialog),Index vector (dialog)  Indices=7:9,1:3  OutputSizes=1,1
  Selector4 : Selector  NumberOfDimensions=2  InputPortWidth=3  IndexOptions=Index vector (dialog),Index vector (dialog)  Indices=1:3,1:3  OutputSizes=1,1
  Selector5 : Selector  NumberOfDimensions=2  InputPortWidth=3  IndexOptions=Index vector (dialog),Index vector (dialog)  Indices=4:6,1:3  OutputSizes=1,1
  Selector6 : Selector  NumberOfDimensions=2  InputPortWidth=3  IndexOptions=Index vector (dialog),Index vector (dialog)  Indices=7:9,1:3  OutputSizes=1,1
  Selector7 : Selector  NumberOfDimensions=2  InputPortWidth=3  IndexOptions=Index vector (dialog),Index vector (dialog)  Indices=10:12,1:3  OutputSizes=1,1
  Selector8 : Selector  NumberOfDimensions=2  InputPortWidth=3  IndexOptions=Index vector (dialog),Index vector (dialog)  Indices=10:12,1:3  OutputSizes=1,1
  To Workspace : ToWorkspace  VariableName=Rp1_0p  SaveFormat=Structure With Time  SampleTime=-1
  To Workspace1 : ToWorkspace  VariableName=Rp2_0p  SaveFormat=Structure With Time  SampleTime=-1
  To Workspace2 : ToWorkspace  VariableName=Rp3_0p  SaveFormat=Structure With Time  SampleTime=-1
  To Workspace3 : ToWorkspace  VariableName=Rp4_0p  SaveFormat=Structure With Time  SampleTime=-1
  To Workspace4 : ToWorkspace  VariableName=Rv1_0p  SaveFormat=Structure With Time  SampleTime=-1
  To Workspace5 : ToWorkspace  VariableName=Rv2_0p  SaveFormat=Structure With Time  SampleTime=-1
  To Workspace6 : ToWorkspace  VariableName=Rv3_0p  SaveFormat=Structure With Time  SampleTime=-1
  To Workspace7 : ToWorkspace  VariableName=Rv4_0p  SaveFormat=Structure With Time  SampleTime=-1
  wires:
  Rp0_W/1 -> Average/1(Rp0_W)
  Rpi_W/1 -> Average/2(Rpi_W)
  Noise Covariance of pi_0 Average/1(Rk_hat) -> Selector4/1, Selector5/1, Selector6/1, Selector7/1
  Average/1(Rpi_0p) -> Noise Covariance of pi_0 Average/1(Rk)
  Selector4/1 -> To Workspace/1
  Selector5/1 -> To Workspace1/1
  Selector6/1 -> To Workspace2/1
  Selector7/1 -> To Workspace3/1
  Rvi_W/1 -> Average/4(Rvi_W)
  Rv0_W/1 -> Average/3(Rv0_W)
  Average/2(Rvi_0p) -> Noise Covariance of vi_0 Average/1(Rk)
  Selector8/1 -> To Workspace7/1
  Selector3/1 -> To Workspace6/1
  Selector2/1 -> To Workspace5/1
  Selector1/1 -> To Workspace4/1
  Noise Covariance of vi_0 Average/1(Rk_hat) -> Selector1/1, Selector2/1, Selector3/1, Selector8/1

== system master_thesis_simulink/Experiments/S1_F2_H2/Experiments ==
  p_0' : Inport
  v_0' : Inport  Port=2
  Selector : Inport  Port=3
  Action Port : ActionPort  ActionPortLabel=if(u1 > 0)
  Constant : Constant  Value=markers_shoulder
  Constant1 : Constant  Value=markers_forearm
  Constant2 : Constant  Value=markers_hand
  EKF : Subsystem
  Human arm : Subsystem  Commented=on
  Human arm_exp : Subsystem  Commented=on
  KF : Subsystem  Commented=on
  LS : Subsystem  Commented=on
  Switch Case : SwitchCase  CaseConditions={0, 1, 2, -1}  ShowDefaultCase=off
  Terminator : Terminator
  tag scope: markers_fo=global, markers_ha=global, markers_sh=global
  wires:
  p_0'/1 -> LS/1(p_0'), EKF/1(p_0'), KF/1(p_0')
  v_0'/1 -> KF/2(v_0'), EKF/2(v_0'), LS/2(v_0')
  Switch Case/1 -> LS/Action
  Switch Case/2 -> KF/Action
  Selector/1 -> Switch Case/1
  [markers_fo] -> LS/4(markers forearm)
  [markers_ha] -> LS/5(markers hand)
  [markers_sh] -> LS/3(markers shoulder)
  [markers_fo] -> EKF/4(markers forearm)
  [markers_ha] -> EKF/5(markers hand)
  [markers_sh] -> EKF/3(markers shoulder)
  Switch Case/4 -> Terminator/1
  Switch Case/3 -> EKF/Action
  Constant1/1 -> [markers_fo]
  Constant/1 -> [markers_sh]
  Constant2/1 -> [markers_ha]

== system master_thesis_simulink/Experiments/S1_F2_H2/Model validation ==
  p_0' : Inport
  Action Port : ActionPort  ActionPortLabel=if(u1 > 0)
  Average : MATLAB Function  TreatAsAtomicUnit=on
  Constant : Constant  Value=zeros(7, 1)
  Display : Subsystem
  Human arm : Subsystem  Commented=on
  Markers_Bases : MATLAB Function  TreatAsAtomicUnit=on
  Mux : Mux  Inputs=3
  Reshape : Reshape  OutputDimensionality=Column vector (2-D)
  Reshape1 : Reshape  OutputDimensionality=Column vector (2-D)
  Scope : Scope
  To Workspace : ToWorkspace  VariableName=markers_Bases  SaveFormat=Structure With Time  SampleTime=-1
  p_0'1 : InportShadow
  p_v__vs_FK_J : MATLAB Function  TreatAsAtomicUnit=on
  wires:
  Markers_Bases/1(markers_shoulder) -> Mux/1, p_v__vs_FK_J/2(shoulder_variables)
  Markers_Bases/2(markers_forearm) -> Reshape1/1, p_v__vs_FK_J/3(forearm_variables)
  Markers_Bases/3(markers_hand) -> Reshape/1, p_v__vs_FK_J/4(hand_variables)
  Constant/1 -> p_v__vs_FK_J/1(q)
  p_0'/1 -> Display/1(p_0')
  Mux/1 -> Scope/1, To Workspace/1
  p_v__vs_FK_J/1(p_Model) -> Display/2(p_FK)
  Reshape/1 -> Mux/3
  Average/1(pk_hat) -> Markers_Bases/1(p_0p_mean)
  p_0'1/1 -> Average/1(pk)
  Reshape1/1 -> Mux/2

== system master_thesis_simulink/Experiments/S1_F2_H2/Noise estimation ==
  Rp0_W : Inport
  Rpi_W : Inport  Port=2
  Rv0_W : Inport  Port=3
  Rvi_W : Inport  Port=4
  Action Port : ActionPort  ActionPortLabel=if(u1 > 0)
  Average : MATLAB Function  TreatAsAtomicUnit=on
  Noise Covariance of pi_0 Average : MATLAB Function  TreatAsAtomicUnit=on
  Noise Covariance of vi_0 Average : MATLAB Function  TreatAsAtomicUnit=on
  Selector1 : Selector  NumberOfDimensions=2  InputPortWidth=3  IndexOptions=Index vector (dialog),Index vector (dialog)  Indices=1:3,1:3  OutputSizes=1,1
  Selector10 : Selector  NumberOfDimensions=2  InputPortWidth=3  IndexOptions=Index vector (dialog),Index vector (dialog)  Indices=13:15,1:3  OutputSizes=1,1
  Selector2 : Selector  NumberOfDimensions=2  InputPortWidth=3  IndexOptions=Index vector (dialog),Index vector (dialog)  Indices=4:6,1:3  OutputSizes=1,1
  Selector3 : Selector  NumberOfDimensions=2  InputPortWidth=3  IndexOptions=Index vector (dialog),Index vector (dialog)  Indices=7:9,1:3  OutputSizes=1,1
  Selector4 : Selector  NumberOfDimensions=2  InputPortWidth=3  IndexOptions=Index vector (dialog),Index vector (dialog)  Indices=1:3,1:3  OutputSizes=1,1
  Selector5 : Selector  NumberOfDimensions=2  InputPortWidth=3  IndexOptions=Index vector (dialog),Index vector (dialog)  Indices=4:6,1:3  OutputSizes=1,1
  Selector6 : Selector  NumberOfDimensions=2  InputPortWidth=3  IndexOptions=Index vector (dialog),Index vector (dialog)  Indices=7:9,1:3  OutputSizes=1,1
  Selector7 : Selector  NumberOfDimensions=2  InputPortWidth=3  IndexOptions=Index vector (dialog),Index vector (dialog)  Indices=10:12,1:3  OutputSizes=1,1
  Selector8 : Selector  NumberOfDimensions=2  InputPortWidth=3  IndexOptions=Index vector (dialog),Index vector (dialog)  Indices=10:12,1:3  OutputSizes=1,1
  Selector9 : Selector  NumberOfDimensions=2  InputPortWidth=3  IndexOptions=Index vector (dialog),Index vector (dialog)  Indices=13:15,1:3  OutputSizes=1,1
  To Workspace : ToWorkspace  VariableName=Rp1_0p  SaveFormat=Structure With Time  SampleTime=-1
  To Workspace1 : ToWorkspace  VariableName=Rp2_0p  SaveFormat=Structure With Time  SampleTime=-1
  To Workspace2 : ToWorkspace  VariableName=Rp3_0p  SaveFormat=Structure With Time  SampleTime=-1
  To Workspace3 : ToWorkspace  VariableName=Rp4_0p  SaveFormat=Structure With Time  SampleTime=-1
  To Workspace4 : ToWorkspace  VariableName=Rv1_0p  SaveFormat=Structure With Time  SampleTime=-1
  To Workspace5 : ToWorkspace  VariableName=Rv2_0p  SaveFormat=Structure With Time  SampleTime=-1
  To Workspace6 : ToWorkspace  VariableName=Rv3_0p  SaveFormat=Structure With Time  SampleTime=-1
  To Workspace7 : ToWorkspace  VariableName=Rv4_0p  SaveFormat=Structure With Time  SampleTime=-1
  To Workspace8 : ToWorkspace  VariableName=Rp5_0p  SaveFormat=Structure With Time  SampleTime=-1
  To Workspace9 : ToWorkspace  VariableName=Rv5_0p  SaveFormat=Structure With Time  SampleTime=-1
  wires:
  Rp0_W/1 -> Average/1(Rp0_W)
  Rpi_W/1 -> Average/2(Rpi_W)
  Average/1(Rpi_0p) -> Noise Covariance of pi_0 Average/1(Rk)
  Selector4/1 -> To Workspace/1
  Selector5/1 -> To Workspace1/1
  Selector6/1 -> To Workspace2/1
  Selector7/1 -> To Workspace3/1
  Rvi_W/1 -> Average/4(Rvi_W)
  Rv0_W/1 -> Average/3(Rv0_W)
  Average/2(Rvi_0p) -> Noise Covariance of vi_0 Average/1(Rk)
  Selector8/1 -> To Workspace7/1
  Selector3/1 -> To Workspace6/1
  Selector2/1 -> To Workspace5/1
  Selector1/1 -> To Workspace4/1
  Selector9/1 -> To Workspace8/1
  Noise Covariance of pi_0 Average/1(Rk_hat) -> Selector4/1, Selector5/1, Selector6/1, Selector7/1, Selector9/1
  Noise Covariance of vi_0 Average/1(Rk_hat) -> Selector1/1, Selector2/1, Selector3/1, Selector8/1, Selector10/1
  Selector10/1 -> To Workspace9/1

== system master_thesis_simulink/Experiments/S2_F0_H2/Experiments ==
  p_0' : Inport
  v_0' : Inport  Port=2
  Selector : Inport  Port=3
  Action Port : ActionPort  ActionPortLabel=if(u1 > 0)
  Constant : Constant  Value=markers_shoulder
  Constant1 : Constant  Value=markers_forearm
  Constant2 : Constant  Value=markers_hand
  EKF : Subsystem
  Human arm : Subsystem  Commented=on
  Human arm_exp : Subsystem  Commented=on
  KF : Subsystem  Commented=on
  LS : Subsystem  Commented=on
  Switch Case : SwitchCase  CaseConditions={0, 1, 2, -1}  ShowDefaultCase=off
  Terminator : Terminator
  tag scope: markers_fo=global, markers_ha=global, markers_sh=global
  wires:
  Constant2/1 -> [markers_ha]
  Constant/1 -> [markers_sh]
  Constant1/1 -> [markers_fo]
  Switch Case/3 -> EKF/Action
  Switch Case/4 -> Terminator/1
  [markers_sh] -> EKF/3(markers shoulder)
  [markers_ha] -> EKF/5(markers hand)
  [markers_fo] -> EKF/4(markers forearm)
  [markers_sh] -> LS/3(markers shoulder)
  [markers_ha] -> LS/5(markers hand)
  [markers_fo] -> LS/4(markers forearm)
  Selector/1 -> Switch Case/1
  Switch Case/2 -> KF/Action
  Switch Case/1 -> LS/Action
  v_0'/1 -> LS/2(v_0'), EKF/2(v_0'), KF/2(v_0')
  p_0'/1 -> KF/1(p_0'), EKF/1(p_0'), LS/1(p_0')

== system master_thesis_simulink/Experiments/S2_F0_H2/Model validation ==
  p_0' : Inport
  Action Port : ActionPort  ActionPortLabel=if(u1 > 0)
  Average : MATLAB Function  TreatAsAtomicUnit=on
  Constant : Constant  Value=zeros(7, 1)
  Display : Subsystem
  Human arm : Subsystem  Commented=on
  Markers_Bases : MATLAB Function  TreatAsAtomicUnit=on
  Mux : Mux  Inputs=3
  Reshape : Reshape  OutputDimensionality=Column vector (2-D)
  Reshape1 : Reshape  OutputDimensionality=Column vector (2-D)
  Scope : Scope
  To Workspace : ToWorkspace  VariableName=markers_Bases  SaveFormat=Structure With Time  SampleTime=-1
  p_0'1 : InportShadow
  p_v__vs_FK_J : MATLAB Function  TreatAsAtomicUnit=on
  wires:
  p_0'1/1 -> Average/1(pk)
  Average/1(pk_hat) -> Markers_Bases/1(p_0p_mean)
  Reshape/1 -> Mux/3
  p_v__vs_FK_J/1(p_Model) -> Display/2(p_FK)
  Mux/1 -> To Workspace/1, Scope/1
  p_0'/1 -> Display/1(p_0')
  Constant/1 -> p_v__vs_FK_J/1(q)
  Markers_Bases/3(markers_hand) -> p_v__vs_FK_J/4(hand_variables), Reshape/1
  Markers_Bases/2(markers_forearm) -> Mux/2, p_v__vs_FK_J/3(forearm_variables)
  Markers_Bases/1(markers_shoulder) -> Reshape1/1, p_v__vs_FK_J/2(shoulder_variables)
  Reshape1/1 -> Mux/1

== system master_thesis_simulink/Experiments/S2_F0_H2/Noise estimation ==
  Rp0_W : Inport
  Rpi_W : Inport  Port=2
  Rv0_W : Inport  Port=3
  Rvi_W : Inport  Port=4
  Action Port : ActionPort  ActionPortLabel=if(u1 > 0)
  Average : MATLAB Function  TreatAsAtomicUnit=on
  Noise Covariance of pi_0 Average : MATLAB Function  TreatAsAtomicUnit=on
  Noise Covariance of vi_0 Average : MATLAB Function  TreatAsAtomicUnit=on
  Selector1 : Selector  NumberOfDimensions=2  InputPortWidth=3  IndexOptions=Index vector (dialog),Index vector (dialog)  Indices=1:3,1:3  OutputSizes=1,1
  Selector2 : Selector  NumberOfDimensions=2  InputPortWidth=3  IndexOptions=Index vector (dialog),Index vector (dialog)  Indices=4:6,1:3  OutputSizes=1,1
  Selector3 : Selector  NumberOfDimensions=2  InputPortWidth=3  IndexOptions=Index vector (dialog),Index vector (dialog)  Indices=7:9,1:3  OutputSizes=1,1
  Selector4 : Selector  NumberOfDimensions=2  InputPortWidth=3  IndexOptions=Index vector (dialog),Index vector (dialog)  Indices=1:3,1:3  OutputSizes=1,1
  Selector5 : Selector  NumberOfDimensions=2  InputPortWidth=3  IndexOptions=Index vector (dialog),Index vector (dialog)  Indices=4:6,1:3  OutputSizes=1,1
  Selector6 : Selector  NumberOfDimensions=2  InputPortWidth=3  IndexOptions=Index vector (dialog),Index vector (dialog)  Indices=7:9,1:3  OutputSizes=1,1
  Selector7 : Selector  NumberOfDimensions=2  InputPortWidth=3  IndexOptions=Index vector (dialog),Index vector (dialog)  Indices=10:12,1:3  OutputSizes=1,1
  Selector8 : Selector  NumberOfDimensions=2  InputPortWidth=3  IndexOptions=Index vector (dialog),Index vector (dialog)  Indices=10:12,1:3  OutputSizes=1,1
  To Workspace : ToWorkspace  VariableName=Rp1_0p  SaveFormat=Structure With Time  SampleTime=-1
  To Workspace1 : ToWorkspace  VariableName=Rp2_0p  SaveFormat=Structure With Time  SampleTime=-1
  To Workspace2 : ToWorkspace  VariableName=Rp3_0p  SaveFormat=Structure With Time  SampleTime=-1
  To Workspace3 : ToWorkspace  VariableName=Rp4_0p  SaveFormat=Structure With Time  SampleTime=-1
  To Workspace4 : ToWorkspace  VariableName=Rv1_0p  SaveFormat=Structure With Time  SampleTime=-1
  To Workspace5 : ToWorkspace  VariableName=Rv2_0p  SaveFormat=Structure With Time  SampleTime=-1
  To Workspace6 : ToWorkspace  VariableName=Rv3_0p  SaveFormat=Structure With Time  SampleTime=-1
  To Workspace7 : ToWorkspace  VariableName=Rv4_0p  SaveFormat=Structure With Time  SampleTime=-1
  wires:
  Noise Covariance of vi_0 Average/1(Rk_hat) -> Selector8/1, Selector3/1, Selector2/1, Selector1/1
  Selector1/1 -> To Workspace4/1
  Selector2/1 -> To Workspace5/1
  Selector3/1 -> To Workspace6/1
  Selector8/1 -> To Workspace7/1
  Average/2(Rvi_0p) -> Noise Covariance of vi_0 Average/1(Rk)
  Rv0_W/1 -> Average/3(Rv0_W)
  Rvi_W/1 -> Average/4(Rvi_W)
  Selector7/1 -> To Workspace3/1
  Selector6/1 -> To Workspace2/1
  Selector5/1 -> To Workspace1/1
  Selector4/1 -> To Workspace/1
  Average/1(Rpi_0p) -> Noise Covariance of pi_0 Average/1(Rk)
  Noise Covariance of pi_0 Average/1(Rk_hat) -> Selector7/1, Selector6/1, Selector5/1, Selector4/1
  Rpi_W/1 -> Average/2(Rpi_W)
  Rp0_W/1 -> Average/1(Rp0_W)
